simulink model "ASM_Traffic_V2X_Complete_Model_2"  (R2019a)
settings: Solver=ode1  StartTime=SIM.tstart.v  StopTime=Inf  FixedStep=SIM.StepSize.v  RelTol=1e-3
PostLoadFcn:
  | if any(exist('dsrtsu_mdlpostloadfcn', 'file') ~= 0), dsrtsu_mdlpostloadfcn('Execute', bdroot); end
  | try, asm_mdl_postloadfcn(bdroot, 'UpdateModel', 2200); catch, disp(lasterr); end,
undefined symbols (not defined in the file): _SensorPnts_1, _SensorPnts_13, _SensorPnts_17, _SensorPnts_21, _SensorPnts_25, _SensorPnts_29, _SensorPnts_33, _SensorPnts_37, _SensorPnts_41, _SensorPnts_45, _SensorPnts_49, _SensorPnts_5, _SensorPnts_53, _SensorPnts_57, _SensorPnts_9, _to_, CPT, G5A, ITS, MDL, rad, s_to_rpm, SIM
libraries: simulink x169, ASM_VehicleDynamics_lib x126, ASM_Traffic_lib x83, ASM_Utils_lib x49, mdbs x45, ASM_Environment_lib x17, dspindex x12, dsaV2xLibraryAux x10, dsmpblib x6, dsaV2xAsn1Library x4, dsaV2xLibrary x4, ASM_BrakeHydraulics_lib x4
(part 31 of 36)

== system ASM_Traffic_V2X_Complete_Model_2/MDLUserInterface/MotionDeskInterface/MOTION_DESK_INTERFACE/Traffic_Animation/Sensors_Animation/Sensor_Points/Line_Sensor_Junction_Shape_Line_Points ==
  ModelSignals : Inport
  Bus Selector : BusSelector  OutputSignals=Pos_x_Junction_Shape_Line_Animation_CoorSys_E,Pos_y_Junction_Shape_Line_Animation_CoorSys_E,Pos_z_Junction_Shape_Line_Animation_CoorSys_E
  CC : Concatenate  NumInputs=4  Mode=Multidimensional array
  Reshape1 : Reshape  OutputDimensionality=Row vector (2-D)
  Reshape2 : Reshape  OutputDimensionality=Row vector (2-D)
  Reshape3 : Reshape  OutputDimensionality=Row vector (2-D)
  zero : Constant  Value=zeros(1,60)  VectorParams1D=off
  AnimationSignals : Outport
  wires:
  zero/1 -> CC/4
  Reshape3/1 -> CC/3
  Reshape2/1 -> CC/2
  Reshape1/1 -> CC/1
  Bus Selector/3 -> Reshape3/1  "<Pos_z_Junction_Shape_Line_Animation_CoorSys_E>"
  Bus Selector/2 -> Reshape2/1  "<Pos_y_Junction_Shape_Line_Animation_CoorSys_E>"
  Bus Selector/1 -> Reshape1/1  "<Pos_x_Junction_Shape_Line_Animation_CoorSys_E>"
  CC/1 -> AnimationSignals/1
  ModelSignals/1 -> Bus Selector/1

== system ASM_Traffic_V2X_Complete_Model_2/MDLUserInterface/MotionDeskInterface/MOTION_DESK_INTERFACE/Traffic_Animation/Sensors_Animation/Sensor_Points/Line_Sensor_Road_Lane_Points ==
  ModelSignals : Inport
  Bus Selector : BusSelector  OutputSignals=Pos_x_Road_Lane_Animation_CoorSys_E,Pos_y_Road_Lane_Animation_CoorSys_E,Pos_z_Road_Lane_Animation_CoorSys_E
  CC : Concatenate  NumInputs=4  Mode=Multidimensional array
  Reshape1 : Reshape  OutputDimensionality=Row vector (2-D)
  Reshape2 : Reshape  OutputDimensionality=Row vector (2-D)
  Reshape3 : Reshape  OutputDimensionality=Row vector (2-D)
  zero : Constant  Value=zeros(1,60)  VectorParams1D=off
  AnimationSignals : Outport
  wires:
  Bus Selector/3 -> Reshape3/1  "<Pos_z_Road_Lane_Animation_CoorSys_E>"
  Bus Selector/2 -> Reshape2/1  "<Pos_y_Road_Lane_Animation_CoorSys_E>"
  Bus Selector/1 -> Reshape1/1  "<Pos_x_Road_Lane_Animation_CoorSys_E>"
  CC/1 -> AnimationSignals/1
  ModelSignals/1 -> Bus Selector/1
  Reshape1/1 -> CC/1
  Reshape2/1 -> CC/2
  Reshape3/1 -> CC/3
  zero/1 -> CC/4

== system ASM_Traffic_V2X_Complete_Model_2/MDLUserInterface/MotionDeskInterface/MOTION_DESK_INTERFACE/Traffic_Animation/Sensors_Animation/Sensor_Points/Line_Sensor_Road_Shape_ContObj_Points ==
  ModelSignals : Inport
  Bus Selector : BusSelector  OutputSignals=Pos_x_Road_Shape_ContObj_Animation_CoorSys_E,Pos_y_Road_Shape_ContObj_Animation_CoorSys_E,Pos_z_Road_Shape_ContObj_Animation_CoorSys_E
  CC : Concatenate  NumInputs=4  Mode=Multidimensional array
  Reshape1 : Reshape  OutputDimensionality=Row vector (2-D)
  Reshape2 : Reshape  OutputDimensionality=Row vector (2-D)
  Reshape3 : Reshape  OutputDimensionality=Row vector (2-D)
  zero : Constant  Value=zeros(1,60)  VectorParams1D=off
  AnimationSignals : Outport
  wires:
  ModelSignals/1 -> Bus Selector/1
  CC/1 -> AnimationSignals/1
  Bus Selector/1 -> Reshape1/1  "<Pos_x_Road_Shape_ContObj_Animation_CoorSys_E>"
  Bus Selector/2 -> Reshape2/1  "<Pos_y_Road_Shape_ContObj_Animation_CoorSys_E>"
  Bus Selector/3 -> Reshape3/1  "<Pos_z_Road_Shape_ContObj_Animation_CoorSys_E>"
  Reshape1/1 -> CC/1
  Reshape2/1 -> CC/2
  Reshape3/1 -> CC/3
  zero/1 -> CC/4

== system ASM_Traffic_V2X_Complete_Model_2/MDLUserInterface/MotionDeskInterface/MOTION_DESK_INTERFACE/Traffic_Animation/Sensors_Animation/Sensor_Points/Line_Sensor_Road_Shape_Line_Points ==
  ModelSignals : Inport
  Bus Selector : BusSelector  OutputSignals=Pos_x_Road_Shape_Line_Animation_CoorSys_E,Pos_y_Road_Shape_Line_Animation_CoorSys_E,Pos_z_Road_Shape_Line_Animation_CoorSys_E
  CC : Concatenate  NumInputs=4  Mode=Multidimensional array
  Reshape1 : Reshape  OutputDimensionality=Row vector (2-D)
  Reshape2 : Reshape  OutputDimensionality=Row vector (2-D)
  Reshape3 : Reshape  OutputDimensionality=Row vector (2-D)
  zero : Constant  Value=zeros(1,60)  VectorParams1D=off
  AnimationSignals : Outport
  wires:
  Bus Selector/3 -> Reshape3/1  "<Pos_z_Road_Shape_Line_Animation_CoorSys_E>"
  Bus Selector/2 -> Reshape2/1  "<Pos_y_Road_Shape_Line_Animation_CoorSys_E>"
  Bus Selector/1 -> Reshape1/1  "<Pos_x_Road_Shape_Line_Animation_CoorSys_E>"
  CC/1 -> AnimationSignals/1
  ModelSignals/1 -> Bus Selector/1
  Reshape1/1 -> CC/1
  Reshape2/1 -> CC/2
  Reshape3/1 -> CC/3
  zero/1 -> CC/4

== system ASM_Traffic_V2X_Complete_Model_2/MDLUserInterface/MotionDeskInterface/MOTION_DESK_INTERFACE/Traffic_Animation/Sensors_Animation/Sensor_Points/Object_Sensor_2D_Points ==
  Transform_In : Inport
  ModelSignals : Inport  Port=2
  Bus Selector1 : BusSelector  OutputSignals=Sensor_1_Front,Sensor_2_Front_Left,Sensor_3_Left,Sensor_4_Rear_Left,Sensor_5_Front_Right,Sensor_6_Right,Sensor_7_Rear_Right
  Bus Selector{2..8} (7 alike) : BusSelector  OutputSignals=Parameters.Pos_Sensor_Apex_CoorSys_V[x;y;z][m],Parameters.Angle_z_Orientation_Sensor_CoorSys_V[deg],SensorOutput.Angle_Hor_Rel[deg],SensorOutput.Distance[m],Parameters.Num_SensorRays_Used[],Parameters.Angle_ScopeZone_Horizontal[deg]  OutputAsBus=on
  Calc_Object_Sensor_2D_Points : Subsystem
  Multiport Switch : MultiPortSwitch  Inputs=7
  Object_Sensor_2D_Transformation : Subsystem
  Saturation : Saturate  UpperLimit=7  LowerLimit=1
  Sensor_Selector : Constant
  AnimationSignals : Outport
  wires:
  Saturation/1 -> Multiport Switch/1
  Bus Selector1/7 -> Bus Selector8/1  "<Sensor_7_Rear_Right>"
  Bus Selector1/6 -> Bus Selector5/1  "<Sensor_6_Right>"
  Bus Selector1/5 -> Bus Selector3/1  "<Sensor_5_Front_Right>"
  Bus Selector1/4 -> Bus Selector2/1  "<Sensor_4_Rear_Left>"
  Bus Selector8/1 -> Multiport Switch/8
  Bus Selector5/1 -> Multiport Switch/7
  Bus Selector3/1 -> Multiport Switch/6
  Bus Selector2/1 -> Multiport Switch/5
  Transform_In/1 -> Object_Sensor_2D_Transformation/1(Transform_In1)
  Object_Sensor_2D_Transformation/1(Transform_Out) -> Calc_Object_Sensor_2D_Points/1(Transform_In)
  Calc_Object_Sensor_2D_Points/1(AnimationSignals) -> AnimationSignals/1
  ModelSignals/1 -> Bus Selector1/1
  Bus Selector1/1 -> Bus Selector4/1  "<Sensor_1_Front>"
  Bus Selector1/2 -> Bus Selector6/1  "<Sensor_2_Front_Left>"
  Bus Selector1/3 -> Bus Selector7/1  "<Sensor_3_Left>"
  Bus Selector7/1 -> Multiport Switch/4
  Bus Selector6/1 -> Multiport Switch/3
  Bus Selector4/1 -> Multiport Switch/2
  Sensor_Selector/1 -> Saturation/1
  Multiport Switch/1 -> Calc_Object_Sensor_2D_Points/2(ModelSignals), Object_Sensor_2D_Transformation/2(ModelSignals)

== system ASM_Traffic_V2X_Complete_Model_2/MDLUserInterface/MotionDeskInterface/MOTION_DESK_INTERFACE/Traffic_Animation/Sensors_Animation/Sensor_Points/Object_Sensor_3D_CustomPoints ==
  ModelSignals : Inport
  Sensor_Selector : Inport  Port=2
  AdaptPointSensor1_To_Dim_60 : Subsystem
  AdaptPointSensor2_To_Dim_60 : Subsystem
  AdaptPointSensor3_To_Dim_60 : Subsystem
  Bus Selector1 : BusSelector  OutputSignals=Sensor_1_Front_Long,Sensor_2_Front_Mid,Sensor_3_Rear
  Bus Selector3 : BusSelector  OutputSignals=ID[],Pos_CoorSys_E[x;y;z][m]
  Bus Selector4 : BusSelector  OutputSignals=CustomPoints.ID[],CustomPoints.Pos_CoorSys_E[x;y;z][m]  OutputAsBus=on
  Bus Selector5 : BusSelector  OutputSignals=ID[],Pos_CoorSys_E[x;y;z][m]
  Bus Selector6 : BusSelector  OutputSignals=CustomPoints.ID[],CustomPoints.Pos_CoorSys_E[x;y;z][m]  OutputAsBus=on
  Bus Selector7 : BusSelector  OutputSignals=CustomPoints.ID[],CustomPoints.Pos_CoorSys_E[x;y;z][m]  OutputAsBus=on
  Bus Selector8 : BusSelector  OutputSignals=ID[],Pos_CoorSys_E[x;y;z][m]
  Compare To Constant3 : simulink/Logic and Bit Operations/Compare To Constant  relop=>  const=-1  OutDataTypeStr=boolean
  DownAway_Dim_3_60 : Constant  Value=[zeros(60*2,1); zeros(60,1)-999999]
  Multiport Switch1 : MultiPortSwitch
  Multiport Switch2 : MultiPortSwitch
  Mux : Mux  Inputs=3
  Reshape_60_3 : Reshape  OutputDimensionality=Customize  OutputDimensions=[60,3]
  Saturation1 : Saturate  UpperLimit=3  LowerLimit=1
  Sw : MultiPortSwitch  DataPortOrder=Zero-based contiguous  Inputs=2  zeroidx=on
  Transpose : Math  Operator=transpose  SaturateOnIntegerOverflow=on
  cc1 : Concatenate  Mode=Multidimensional array
  zero_60 : Constant  Value=zeros(1,60)  VectorParams1D=off
  AnimationSignals : Outport
  wires:
  cc1/1 -> AnimationSignals/1
  zero_60/1 -> cc1/2
  AdaptPointSensor3_To_Dim_60/1(ID_Adatpted[]) -> Multiport Switch2/4
  AdaptPointSensor3_To_Dim_60/2(Pos_ObjectPoint_CoorSys_E_Adapted[x;y;z][m]) -> Multiport Switch1/4
  Multiport Switch1/1 -> Sw/3
  Bus Selector8/2 -> AdaptPointSensor3_To_Dim_60/2(Pos_ObjectPoint_CoorSys_E[x;y;z][m])  "<Pos_CoorSys_E[x;y;z][m]>"
  Bus Selector5/2 -> AdaptPointSensor2_To_Dim_60/2(Pos_ObjectPoint_CoorSys_E[x;y;z][m])  "<Pos_CoorSys_E[x;y;z][m]>"
  Bus Selector5/1 -> AdaptPointSensor2_To_Dim_60/1(ID[])  "<ID[]>"
  Bus Selector1/1 -> Bus Selector4/1  "<Sensor_1_Front_Long>"
  Bus Selector1/2 -> Bus Selector6/1  "<Sensor_2_Front_Mid>"
  Bus Selector1/3 -> Bus Selector7/1  "<Sensor_3_Rear>"
  Multiport Switch2/1 -> Compare To Constant3/1
  Reshape_60_3/1 -> Transpose/1
  Bus Selector6/1 -> Bus Selector5/1
  Bus Selector7/1 -> Bus Selector8/1
  Bus Selector3/1 -> AdaptPointSensor1_To_Dim_60/1(ID[])  "<ID[]>"
  Bus Selector3/2 -> AdaptPointSensor1_To_Dim_60/2(Pos_ObjectPoint_CoorSys_E[x;y;z][m])  "<Pos_CoorSys_E[x;y;z][m]>"
  Bus Selector4/1 -> Bus Selector3/1
  AdaptPointSensor1_To_Dim_60/1(ID_Adatpted[]) -> Multiport Switch2/2
  AdaptPointSensor1_To_Dim_60/2(Pos_ObjectPoint_CoorSys_E_Adapted[x;y;z][m]) -> Multiport Switch1/2
  Bus Selector8/1 -> AdaptPointSensor3_To_Dim_60/1(ID[])  "<ID[]>"
  ModelSignals/1 -> Bus Selector1/1
  Mux/1 -> Sw/1
  Compare To Constant3/1 -> Mux/3, Mux/2, Mux/1
  Sensor_Selector/1 -> Saturation1/1
  DownAway_Dim_3_60/1 -> Sw/2
  Saturation1/1 -> Multiport Switch1/1, Multiport Switch2/1
  Sw/1 -> Reshape_60_3/1
  Transpose/1 -> cc1/1
  AdaptPointSensor2_To_Dim_60/2(Pos_ObjectPoint_CoorSys_E_Adapted[x;y;z][m]) -> Multiport Switch1/3
  AdaptPointSensor2_To_Dim_60/1(ID_Adatpted[]) -> Multiport Switch2/3

== system ASM_Traffic_V2X_Complete_Model_2/MDLUserInterface/MotionDeskInterface/MOTION_DESK_INTERFACE/Traffic_Animation/Sensors_Animation/Sensor_Points/Object_Sensor_3D_Points ==
  ModelSignals : Inport
  Sensor_Selector : Inport  Port=2
  Bus Selector1 : BusSelector  OutputSignals=Sensor_1_Front_Long,Sensor_2_Front_Mid,Sensor_3_Rear
  Bus Selector2 : BusSelector  OutputSignals=Flag_NearestPnt_Occluded[-1|0|1],Flag_Object_In_Scope[0Out|1In],Pos_Object_NearestPnt_E[x;y;z][m]
  Bus Selector4 : BusSelector  OutputSignals=SensorOutput.Pos_Object_NearestPnt_E[x;y;z][m],Info.Flag_Object_In_Scope[0Out|1In],SensorOutput.Flag_NearestPnt_Occluded[-1|0|1]  OutputAsBus=on
  Bus Selector6 : BusSelector  OutputSignals=SensorOutput.Pos_Object_NearestPnt_E[x;y;z][m],Info.Flag_Object_In_Scope[0Out|1In],SensorOutput.Flag_NearestPnt_Occluded[-1|0|1]  OutputAsBus=on
  Bus Selector7 : BusSelector  OutputSignals=SensorOutput.Pos_Object_NearestPnt_E[x;y;z][m],Info.Flag_Object_In_Scope[0Out|1In],SensorOutput.Flag_NearestPnt_Occluded[-1|0|1]  OutputAsBus=on
  DownAway : Constant  Value=[zeros(MDL.Traffic.Sensors.ObjectSensor3D_Calculation.Const_Sensor_Output_Dimension.v*2,1); zeros(MDL.Traffic.Sensors.ObjectSensor3D_Calculation.Const_Sensor_Output_Dimension.v,1)-999999]
  DownAway1 : Constant  Value=[zeros(2,60-MDL.Traffic.Sensors.ObjectSensor3D_Calculation.Const_Sensor_Output_Dimension.v); zeros(1,60-MDL.Traffic.Sensors.ObjectSensor3D_Calculation.Const_Sensor_Output_Dimension.v)-999999]
  Hide_Occluded_NearestPoint[0|1] : Constant  Value=0
  Ignore_Negative : RelationalOperator  Operator===  RndMeth=Simplest
  Mask_Hidden_Objects : Product
  Multiport Switch : MultiPortSwitch
  Mux : Mux  Inputs=3
  Negate : Sum  Inputs=+-
  Product : Product
  Reshape1 : Reshape  OutputDimensionality=Customize  OutputDimensions=[MDL.Traffic.Sensors.ObjectSensor3D_Calculation.Const_Sensor_Output_Dimension.v,3]
  Saturation : Saturate  UpperLimit=3  LowerLimit=1
  Saturation1 : Saturate  UpperLimit=1  LowerLimit=0
  Show_Occluded_NearestPoint[0|1]1 : Constant
  Show_Occluded_NearestPoint[0|1]2 : Constant
  Sw : MultiPortSwitch  DataPortOrder=Zero-based contiguous  Inputs=2  zeroidx=on
  Transpose : Math  Operator=transpose  SaturateOnIntegerOverflow=on
  cc : Concatenate  Mode=Multidimensional array  ConcatenateDimension=2
  cc1 : Concatenate  Mode=Multidimensional array
  zero3 : Constant  Value=zeros(1,60)  VectorParams1D=off
  AnimationSignals : Outport
  wires:
  Mask_Hidden_Objects/1 -> Mux/2, Mux/1, Mux/3
  Negate/1 -> Mask_Hidden_Objects/1
  Bus Selector2/2 -> Mask_Hidden_Objects/2  "<Flag_Object_In_Scope[0Out|1In]>"
  Ignore_Negative/1 -> Product/2
  Show_Occluded_NearestPoint[0|1]2/1 -> Ignore_Negative/2
  Bus Selector2/1 -> Ignore_Negative/1  "<Flag_NearestPnt_Occluded[-1|0|1]>"
  Show_Occluded_NearestPoint[0|1]1/1 -> Negate/1
  Product/1 -> Negate/2
  Mux/1 -> Sw/1
  Saturation1/1 -> Product/1
  Hide_Occluded_NearestPoint[0|1]/1 -> Saturation1/1
  Saturation/1 -> Multiport Switch/1
  ModelSignals/1 -> Bus Selector1/1
  Bus Selector1/1 -> Bus Selector4/1  "<Sensor_1_Front_Long>"
  Bus Selector1/2 -> Bus Selector6/1  "<Sensor_2_Front_Mid>"
  Bus Selector1/3 -> Bus Selector7/1  "<Sensor_3_Rear>"
  Bus Selector7/1 -> Multiport Switch/4
  Bus Selector6/1 -> Multiport Switch/3
  Bus Selector4/1 -> Multiport Switch/2
  Sensor_Selector/1 -> Saturation/1
  Multiport Switch/1 -> Bus Selector2/1
  Bus Selector2/3 -> Sw/3  "<Pos_Object_NearestPnt_E[x;y;z][m]>"
  DownAway/1 -> Sw/2
  Sw/1 -> Reshape1/1
  Reshape1/1 -> Transpose/1
  Transpose/1 -> cc/1
  DownAway1/1 -> cc/2
  cc/1 -> cc1/1
  zero3/1 -> cc1/2
  cc1/1 -> AnimationSignals/1

== system ASM_Traffic_V2X_Complete_Model_2/MDLUserInterface/MotionDeskInterface/MOTION_DESK_INTERFACE/Traffic_Animation/Sensors_Animation/Sensor_Points/Object_Sensor_3D_RadarEffect_Points ==
  ModelSignals : Inport
  Sensor_Selector : Inport  Port=2
  AdaptPointDimensionSensor1 : Subsystem
  AdaptPointDimensionSensor2 : Subsystem
  AdaptPointDimensionSensor3 : Subsystem
  Bus Selector1 : BusSelector  OutputSignals=Sensor_1_Front_Long,Sensor_2_Front_Mid,Sensor_3_Rear
  Bus Selector3 : BusSelector  OutputSignals=ID[],Pos_ObjectPoint_CoorSys_E[x;y;z][m]
  Bus Selector4 : BusSelector  OutputSignals=RadarEffects.ID[],RadarEffects.Pos_ObjectPoint_CoorSys_E[x;y;z][m]  OutputAsBus=on
  Bus Selector5 : BusSelector  OutputSignals=ID[],Pos_ObjectPoint_CoorSys_E[x;y;z][m]
  Bus Selector6 : BusSelector  OutputSignals=RadarEffects.ID[],RadarEffects.Pos_ObjectPoint_CoorSys_E[x;y;z][m]  OutputAsBus=on
  Bus Selector7 : BusSelector  OutputSignals=RadarEffects.ID[],RadarEffects.Pos_ObjectPoint_CoorSys_E[x;y;z][m]  OutputAsBus=on
  Bus Selector8 : BusSelector  OutputSignals=ID[],Pos_ObjectPoint_CoorSys_E[x;y;z][m]
  Compare To Constant3 : simulink/Logic and Bit Operations/Compare To Constant  relop=>  const=-1  OutDataTypeStr=boolean
  DownAway : Constant  Value=[zeros(60*2,1); zeros(60,1)-999999]
  Multiport Switch1 : MultiPortSwitch
  Multiport Switch2 : MultiPortSwitch
  Mux : Mux  Inputs=3
  Reshape1 : Reshape  OutputDimensionality=Customize  OutputDimensions=[60,3]
  Saturation1 : Saturate  UpperLimit=3  LowerLimit=1
  Sw : MultiPortSwitch  DataPortOrder=Zero-based contiguous  Inputs=2  zeroidx=on
  Transpose : Math  Operator=transpose  SaturateOnIntegerOverflow=on
  cc1 : Concatenate  Mode=Multidimensional array
  zero3 : Constant  Value=zeros(1,60)  VectorParams1D=off
  AnimationSignals : Outport
  wires:
  Bus Selector8/2 -> AdaptPointDimensionSensor3/2(Pos_ObjectPoint_CoorSys_E[x;y;z][m])  "<Pos_ObjectPoint_CoorSys_E[x;y;z][m]>"
  cc1/1 -> AnimationSignals/1
  zero3/1 -> cc1/2
  Transpose/1 -> cc1/1
  Reshape1/1 -> Transpose/1
  Mux/1 -> Sw/1
  Sw/1 -> Reshape1/1
  DownAway/1 -> Sw/2
  Compare To Constant3/1 -> Mux/1, Mux/2, Mux/3
  AdaptPointDimensionSensor3/2(Pos_ObjectPoint_CoorSys_E_Adapted[x;y;z][m]) -> Multiport Switch1/4
  AdaptPointDimensionSensor3/1(ID_Adatpted[]) -> Multiport Switch2/4
  Bus Selector5/2 -> AdaptPointDimensionSensor2/2(Pos_ObjectPoint_CoorSys_E[x;y;z][m])  "<Pos_ObjectPoint_CoorSys_E[x;y;z][m]>"
  AdaptPointDimensionSensor2/2(Pos_ObjectPoint_CoorSys_E_Adapted[x;y;z][m]) -> Multiport Switch1/3
  AdaptPointDimensionSensor2/1(ID_Adatpted[]) -> Multiport Switch2/3
  AdaptPointDimensionSensor1/2(Pos_ObjectPoint_CoorSys_E_Adapted[x;y;z][m]) -> Multiport Switch1/2
  AdaptPointDimensionSensor1/1(ID_Adatpted[]) -> Multiport Switch2/2
  Bus Selector3/2 -> AdaptPointDimensionSensor1/2(Pos_ObjectPoint_CoorSys_E[x;y;z][m])  "<Pos_ObjectPoint_CoorSys_E[x;y;z][m]>"
  Bus Selector3/1 -> AdaptPointDimensionSensor1/1(ID[])  "<ID[]>"
  Multiport Switch1/1 -> Sw/3
  Multiport Switch2/1 -> Compare To Constant3/1
  Bus Selector8/1 -> AdaptPointDimensionSensor3/1(ID[])  "<ID[]>"
  Bus Selector5/1 -> AdaptPointDimensionSensor2/1(ID[])  "<ID[]>"
  Sensor_Selector/1 -> Saturation1/1
  Saturation1/1 -> Multiport Switch2/1, Multiport Switch1/1
  ModelSignals/1 -> Bus Selector1/1
  Bus Selector1/1 -> Bus Selector4/1  "<Sensor_1_Front_Long>"
  Bus Selector1/2 -> Bus Selector6/1  "<Sensor_2_Front_Mid>"
  Bus Selector1/3 -> Bus Selector7/1  "<Sensor_3_Rear>"
  Bus Selector7/1 -> Bus Selector8/1
  Bus Selector6/1 -> Bus Selector5/1
  Bus Selector4/1 -> Bus Selector3/1

== system ASM_Traffic_V2X_Complete_Model_2/MDLUserInterface/MotionDeskInterface/MOTION_DESK_INTERFACE/Traffic_Animation/Sensors_Animation/Sensor_Points/Sensor_Points ==
  AnimationSignals : Inport
  MD_Object1 : mdbs/MD_Object  strObjId=23  strObjName=_SensorPnts_1-4  strBlockType=OBJ  bGUIEventOK=0
      settings: SourceProductName=dSPACE MotionDesk Blockset
  MD_Object10 : mdbs/MD_Object  strObjId=32  strObjName=_SensorPnts_37-40  strBlockType=OBJ  bGUIEventOK=0
      settings: SourceProductName=dSPACE MotionDesk Blockset
  MD_Object11 : mdbs/MD_Object  strObjId=35  strObjName=_SensorPnts_49-52  strBlockType=OBJ  bGUIEventOK=0
      settings: SourceProductName=dSPACE MotionDesk Blockset
  MD_Object13 : mdbs/MD_Object  strObjId=33  strObjName=_SensorPnts_41-44  strBlockType=OBJ  bGUIEventOK=0
      settings: SourceProductName=dSPACE MotionDesk Blockset
  MD_Object14 : mdbs/MD_Object  strObjId=34  strObjName=_SensorPnts_45-48  strBlockType=OBJ  bGUIEventOK=0
      settings: SourceProductName=dSPACE MotionDesk Blockset
  MD_Object15 : mdbs/MD_Object  strObjId=36  strObjName=_SensorPnts_53-56  strBlockType=OBJ  bGUIEventOK=0
      settings: SourceProductName=dSPACE MotionDesk Blockset
  MD_Object16 : mdbs/MD_Object  strObjId=37  strObjName=_SensorPnts_57-60  strBlockType=OBJ  bGUIEventOK=0
      settings: SourceProductName=dSPACE MotionDesk Blockset
  MD_Object2 : mdbs/MD_Object  strObjId=24  strObjName=_SensorPnts_5-8  strBlockType=OBJ  bGUIEventOK=0
      settings: SourceProductName=dSPACE MotionDesk Blockset
  MD_Object3 : mdbs/MD_Object  strObjId=25  strObjName=_SensorPnts_9-12  strBlockType=OBJ  bGUIEventOK=0
      settings: SourceProductName=dSPACE MotionDesk Blockset
  MD_Object4 : mdbs/MD_Object  strObjId=26  strObjName=_SensorPnts_13-16  strBlockType=OBJ  bGUIEventOK=0
      settings: SourceProductName=dSPACE MotionDesk Blockset
  MD_Object5 : mdbs/MD_Object  strObjId=27  strObjName=_SensorPnts_17-20  strBlockType=OBJ  bGUIEventOK=0
      settings: SourceProductName=dSPACE MotionDesk Blockset
  MD_Object6 : mdbs/MD_Object  strObjId=28  strObjName=_SensorPnts_21-24  strBlockType=OBJ  bGUIEventOK=0
      settings: SourceProductName=dSPACE MotionDesk Blockset
  MD_Object7 : mdbs/MD_Object  strObjId=29  strObjName=_SensorPnts_25-28  strBlockType=OBJ  bGUIEventOK=0
      settings: SourceProductName=dSPACE MotionDesk Blockset
  MD_Object8 : mdbs/MD_Object  strObjId=30  strObjName=_SensorPnts_29-32  strBlockType=OBJ  bGUIEventOK=0
      settings: SourceProductName=dSPACE MotionDesk Blockset
  MD_Object9 : mdbs/MD_Object  strObjId=31  strObjName=_SensorPnts_33-36  strBlockType=OBJ  bGUIEventOK=0
      settings: SourceProductName=dSPACE MotionDesk Blockset
  Selector : Selector  NumberOfDimensions=2  IndexMode=Zero-based  InputPortWidth=15  IndexOptions=Index vector (dialog),Index vector (dialog)  Indices=-1,[0:3]  OutputSizes=1,1
  Selector1 : Selector  NumberOfDimensions=2  IndexMode=Zero-based  InputPortWidth=15  IndexOptions=Index vector (dialog),Index vector (dialog)  Indices=-1,[0:3]+4  OutputSizes=1,1
  Selector10 : Selector  NumberOfDimensions=2  IndexMode=Zero-based  InputPortWidth=15  IndexOptions=Index vector (dialog),Index vector (dialog)  Indices=-1,[0:3]+52  OutputSizes=1,1
  Selector12 : Selector  NumberOfDimensions=2  IndexMode=Zero-based  InputPortWidth=15  IndexOptions=Index vector (dialog),Index vector (dialog)  Indices=-1,[0:3]+40  OutputSizes=1,1
  Selector13 : Selector  NumberOfDimensions=2  IndexMode=Zero-based  InputPortWidth=15  IndexOptions=Index vector (dialog),Index vector (dialog)  Indices=-1,[0:3]+44  OutputSizes=1,1
  Selector14 : Selector  NumberOfDimensions=2  IndexMode=Zero-based  InputPortWidth=15  IndexOptions=Index vector (dialog),Index vector (dialog)  Indices=-1,[0:3]+56  OutputSizes=1,1
  Selector15 : Selector  NumberOfDimensions=2  IndexMode=Zero-based  InputPortWidth=15  IndexOptions=Index vector (dialog),Index vector (dialog)  Indices=-1,[0:3]+48  OutputSizes=1,1
  Selector2 : Selector  NumberOfDimensions=2  IndexMode=Zero-based  InputPortWidth=15  IndexOptions=Index vector (dialog),Index vector (dialog)  Indices=-1,[0:3]+8  OutputSizes=1,1
  Selector3 : Selector  NumberOfDimensions=2  IndexMode=Zero-based  InputPortWidth=15  IndexOptions=Index vector (dialog),Index vector (dialog)  Indices=-1,[0:3]+12  OutputSizes=1,1
  Selector4 : Selector  NumberOfDimensions=2  IndexMode=Zero-based  InputPortWidth=15  IndexOptions=Index vector (dialog),Index vector (dialog)  Indices=-1,[0:3]+16  OutputSizes=1,1
  Selector5 : Selector  NumberOfDimensions=2  IndexMode=Zero-based  InputPortWidth=15  IndexOptions=Index vector (dialog),Index vector (dialog)  Indices=-1,[0:3]+20  OutputSizes=1,1
  Selector6 : Selector  NumberOfDimensions=2  IndexMode=Zero-based  InputPortWidth=15  IndexOptions=Index vector (dialog),Index vector (dialog)  Indices=-1,[0:3]+24  OutputSizes=1,1
  Selector7 : Selector  NumberOfDimensions=2  IndexMode=Zero-based  InputPortWidth=15  IndexOptions=Index vector (dialog),Index vector (dialog)  Indices=-1,[0:3]+28  OutputSizes=1,1
  Selector8 : Selector  NumberOfDimensions=2  IndexMode=Zero-based  InputPortWidth=15  IndexOptions=Index vector (dialog),Index vector (dialog)  Indices=-1,[0:3]+32  OutputSizes=1,1
  Selector9 : Selector  NumberOfDimensions=2  IndexMode=Zero-based  InputPortWidth=15  IndexOptions=Index vector (dialog),Index vector (dialog)  Indices=-1,[0:3]+36  OutputSizes=1,1
  Terminator{1..11,13..16} (15 alike) : Terminator
  wires:
  Selector8/1 -> MD_Object9/1
  Selector7/1 -> MD_Object8/1
  Selector6/1 -> MD_Object7/1
  Selector5/1 -> MD_Object6/1
  Selector4/1 -> MD_Object5/1
  Selector3/1 -> MD_Object4/1
  MD_Object9/1 -> Terminator9/1
  Selector2/1 -> MD_Object3/1
  Selector1/1 -> MD_Object2/1
  Selector/1 -> MD_Object1/1
  MD_Object8/1 -> Terminator8/1
  MD_Object7/1 -> Terminator7/1
  MD_Object6/1 -> Terminator6/1
  MD_Object5/1 -> Terminator5/1
  MD_Object4/1 -> Terminator4/1
  MD_Object3/1 -> Terminator3/1
  MD_Object2/1 -> Terminator2/1
  MD_Object1/1 -> Terminator1/1
  MD_Object10/1 -> Terminator10/1
  Selector9/1 -> MD_Object10/1
  MD_Object13/1 -> Terminator13/1
  Selector12/1 -> MD_Object13/1
  MD_Object14/1 -> Terminator14/1
  Selector13/1 -> MD_Object14/1
  AnimationSignals/1 -> Selector/1, Selector15/1, Selector10/1, Selector14/1, Selector13/1, Selector12/1, Selector9/1, Selector8/1, Selector7/1, Selector6/1, Selector5/1, Selector4/1, Selector3/1, Selector2/1, Selector1/1
  MD_Object15/1 -> Terminator11/1
  Selector10/1 -> MD_Object15/1
  MD_Object16/1 -> Terminator15/1
  Selector14/1 -> MD_Object16/1
  Selector15/1 -> MD_Object11/1
  MD_Object11/1 -> Terminator16/1

== system ASM_Traffic_V2X_Complete_Model_2/MDLUserInterface/MotionDeskInterface/MOTION_DESK_INTERFACE/Traffic_Animation/Sensors_Animation/Sensor_Points/Traffic_Sign_Sensor_Points ==
  ModelSignals : Inport
  Bus Selector2 : BusSelector  OutputSignals=Sensor_Front_1.SensorOutput[].Traffic_Sign_Valid[0|1],Sensor_Front_1.SensorOutput[].Pos_CoorSys_E[x;y;z][m]
  DownAway : Constant  Value=[zeros(2,MDL.Traffic.Sensors.TrafficSignSensorDyn_Calculation.Const_Sensor_Output_Dimension.v); zeros(1,MDL.Traffic.Sensors.TrafficSignSensorDyn_Calculation.Const_Sensor_Output_Dimension.v)-999999]
  DownAway1 : Constant  Value=[zeros(2,60-MDL.Traffic.Sensors.TrafficSignSensorDyn_Calculation.Const_Sensor_Output_Dimension.v); zeros(1,60-MDL.Traffic.Sensors.TrafficSignSensorDyn_Calculation.Const_Sensor_Output_Dimension.v)-999999]
  Reshape1 : Reshape  OutputDimensionality=Customize  OutputDimensions=[3,MDL.Traffic.Sensors.TrafficSignSensorDyn_Calculation.Const_Sensor_Output_Dimension.v]
  Sw : MultiPortSwitch  DataPortOrder=Zero-based contiguous  Inputs=2  zeroidx=on
  Trans : Math  Operator=transpose  SaturateOnIntegerOverflow=on
  cc : Concatenate  NumInputs=3  Mode=Multidimensional array  ConcatenateDimension=2
  cc1 : Concatenate  Mode=Multidimensional array  ConcatenateDimension=2
  cc2 : Concatenate  Mode=Multidimensional array
  zero3 : Constant  Value=zeros(1,60)  VectorParams1D=off
  AnimationSignals : Outport
  wires:
  cc2/1 -> AnimationSignals/1
  cc1/1 -> cc2/1
  zero3/1 -> cc2/2
  Sw/1 -> cc1/1
  DownAway1/1 -> cc1/2
  DownAway/1 -> Sw/2
  Trans/1 -> Sw/1
  cc/1 -> Trans/1
  Reshape1/1 -> Sw/3
  Bus Selector2/1 -> cc/2, cc/1, cc/3  "<Traffic_Sign_Valid[0|1]>"
  Bus Selector2/2 -> Reshape1/1  "<Pos_CoorSys_E[x;y;z][m]>"
  ModelSignals/1 -> Bus Selector2/1

== system ASM_Traffic_V2X_Complete_Model_2/IO/I//O_Subsystem/Bus Configuration (1) - In/Simulated ECUs/DrivekitCAN/Drivekit/TX/PDUs ==
  Input : Inport
  BRAKE_REPORT : Subsystem
  Bus Selector : BusSelector  OutputSignals=signal3.Lat Value,signal3.Long Value,signal3.Heading Value,CurrentLane
  CHASSIS_CONTROL_REPORT : Subsystem
  ESP12 : Subsystem
  FAULT_REPORT : Subsystem
  GPS_HEADING : Subsystem
  GPS_LAT : Subsystem
  GPS_LONG : Subsystem
  LANE_REPORT : Subsystem
  SAS11 : Subsystem
  STEERING_ANGLE_REPORT : Subsystem
  STEERING_REPORT : Subsystem
  THROTTLE_REPORT : Subsystem
  WHL_SPD11 : Subsystem
  _PDUs_ : BusCreator  Inputs=13
  PDUs : Outport
  wires:
  _PDUs_/1 -> PDUs/1  "PDUs"
  SAS11/1(SAS11) -> _PDUs_/1  "SAS11"
  WHL_SPD11/1(WHL_SPD11) -> _PDUs_/2  "WHL_SPD11"
  ESP12/1(ESP12) -> _PDUs_/3  "ESP12"
  BRAKE_REPORT/1(BRAKE_REPORT) -> _PDUs_/4  "BRAKE_REPORT"
  STEERING_REPORT/1(STEERING_REPORT) -> _PDUs_/5  "STEERING_REPORT"
  THROTTLE_REPORT/1(THROTTLE_REPORT) -> _PDUs_/6  "THROTTLE_REPORT"
  FAULT_REPORT/1(FAULT_REPORT) -> _PDUs_/7  "FAULT_REPORT"
  STEERING_ANGLE_REPORT/1(STEERING_ANGLE_REPORT) -> _PDUs_/8  "STEERING_ANGLE_REPORT"
  CHASSIS_CONTROL_REPORT/1(CHASSIS_CONTROL_REPORT) -> _PDUs_/9  "CHASSIS_CONTROL_REPORT"
  GPS_LAT/1(GPS_LAT) -> _PDUs_/10  "GPS_LAT"
  GPS_LONG/1(GPS_LONG) -> _PDUs_/11  "GPS_LONG"
  GPS_HEADING/1(GPS_HEADING) -> _PDUs_/12  "GPS_HEADING"
  LANE_REPORT/1(LANE_REPORT) -> _PDUs_/13  "LANE_REPORT"
  Input/1 -> SAS11/1(Input), Bus Selector/1, WHL_SPD11/1(Input)
  Bus Selector/1 -> GPS_LAT/1(Input)  "<Lat Value>"
  Bus Selector/2 -> GPS_LONG/1(Input)  "<Long Value>"
  Bus Selector/3 -> GPS_HEADING/1(Input)  "<Heading Value>"
  Bus Selector/4 -> LANE_REPORT/1(Input)  "<CurrentLane>"

== system ASM_Traffic_V2X_Complete_Model_2/IO/I//O_Subsystem/Bus Configuration (1) - Out/Simulated ECUs/DrivekitCAN/Drivekit/RX/PDUs ==
  PDUs : Inport
  BRAKE_COMMAND : Subsystem
  BRAKE_DISABLE : Subsystem
  BRAKE_ENABLE : Subsystem
  CHASSIS_CONTROL_COMMAND : Subsystem
  STEERING_ANGLE_COMMAND : Subsystem
  STEERING_DISABLE : Subsystem
  STEERING_ENABLE : Subsystem
  STEERING_TORQUE_COMMAND : Subsystem
  THROTTLE_COMMAND : Subsystem
  THROTTLE_DISABLE : Subsystem
  THROTTLE_ENABLE : Subsystem
  _PDUs_ : BusSelector  OutputSignals=BRAKE_ENABLE,BRAKE_DISABLE,BRAKE_COMMAND,STEERING_ENABLE,STEERING_DISABLE,STEERING_TORQUE_COMMAND,THROTTLE_ENABLE,THROTTLE_DISABLE,THROTTLE_COMMAND,STEERING_ANGLE_COMMAND,CHASSIS_CONTROL_COMMAND
  wires:
  PDUs/1 -> _PDUs_/1  "PDUs"
  _PDUs_/1 -> BRAKE_ENABLE/1(BRAKE_ENABLE)  "<BRAKE_ENABLE>"
  _PDUs_/2 -> BRAKE_DISABLE/1(BRAKE_DISABLE)  "<BRAKE_DISABLE>"
  _PDUs_/3 -> BRAKE_COMMAND/1(BRAKE_COMMAND)  "<BRAKE_COMMAND>"
  _PDUs_/4 -> STEERING_ENABLE/1(STEERING_ENABLE)  "<STEERING_ENABLE>"
  _PDUs_/5 -> STEERING_DISABLE/1(STEERING_DISABLE)  "<STEERING_DISABLE>"
  _PDUs_/6 -> STEERING_TORQUE_COMMAND/1(STEERING_TORQUE_COMMAND)  "<STEERING_TORQUE_COMMAND>"
  _PDUs_/7 -> THROTTLE_ENABLE/1(THROTTLE_ENABLE)  "<THROTTLE_ENABLE>"
  _PDUs_/8 -> THROTTLE_DISABLE/1(THROTTLE_DISABLE)  "<THROTTLE_DISABLE>"
  _PDUs_/9 -> THROTTLE_COMMAND/1(THROTTLE_COMMAND)  "<THROTTLE_COMMAND>"
  _PDUs_/10 -> STEERING_ANGLE_COMMAND/1(STEERING_ANGLE_COMMAND)  "<STEERING_ANGLE_COMMAND>"
  _PDUs_/11 -> CHASSIS_CONTROL_COMMAND/1(CHASSIS_CONTROL_COMMAND)  "<CHASSIS_CONTROL_COMMAND>"

== system ASM_Traffic_V2X_Complete_Model_2/MDL/Environment/Traffic/Sensors/Object_Sensor_3D/CustomPoints/Sensor1/CustomPoints ==
  Sensor_Idx[] : Inport
  Sensor_Data[] : Inport  Port=2
  Enable : EnablePort
  Bus Creator2 : BusCreator  Inputs=17
  CUSTOM_POINTS_1 : ASM_Traffic_lib/Sensors/Custom Points/CUSTOM_POINTS  Tag=ASM_SUBCOMPONENT  Sw_Visible_Points_Filter_Enable=MDL.Traffic.Sensors.CustomPoints_1.Sw_Visible_Points_Filter_Enable  Sw_Sort_Enable=MDL.Traffic.Sensors.CustomPoints_1.Sw_Sort_Enable  Sw_Sort_Attribute=MDL.Traffic.Sensors.CustomPoints_1.Sw_Sort_Attribute  Sw_Sort_Direction=MDL.Traffic.Sensors.CustomPoints_1.Sw_Sort_Direction  ASMProperties=struct('Name','CUSTOM_POINTS','Version','1.0','Library','ASM_Traffic_lib')  ASMInstanceName=custom_points  ASMInstanceID=1  Const_Output_Dimension_Objects=MDL.Traffic.Sensors.CustomPoints_1.Const_Output_Dimension_Objects  Const_Output_Dimension_Object_Points=MDL.Traffic.Sensors.CustomPoints_1.Const_Output_Dimension_Object_Points
  MODELDESK_GROUP : ASM_Utils_lib/ModelDeskInterface/MODELDESK_GROUP  MDLDGroup=Object Sensor 3D 1  ASMProperties=struct('Name','MODELDESK_GROUP','Version','1.0','Library','ASM_Utils_lib')
  Terminator : Terminator
  CustomPoint_Signals[] : Outport  OutputWhenDisabled=reset  InitialOutput=[0]
  wires:
  CUSTOM_POINTS_1/18 -> Bus Creator2/17  "Object_Type[]"
  CUSTOM_POINTS_1/7 -> Bus Creator2/6  "a_CoorSys_S[m|s2]"
  CUSTOM_POINTS_1/11 -> Bus Creator2/10  "Angle_Ver_CoorSys_S[deg]"
  CUSTOM_POINTS_1/8 -> Bus Creator2/7  "Pos_CoorSys_S[x;y;z][m]"
  CUSTOM_POINTS_1/9 -> Bus Creator2/8  "Pos_CoorSys_E[x;y;z][m]"
  CUSTOM_POINTS_1/15 -> Bus Creator2/14  "Data_4[]"
  CUSTOM_POINTS_1/16 -> Bus Creator2/15  "Data_5[]"
  CUSTOM_POINTS_1/14 -> Bus Creator2/13  "Data_3[]"
  CUSTOM_POINTS_1/2 -> Bus Creator2/1  "Flag_In_Scope[0|1]"
  CUSTOM_POINTS_1/6 -> Bus Creator2/5  "v_CoorSys_S[m|s]"
  CUSTOM_POINTS_1/17 -> Bus Creator2/16  "Object_ID[]"
  CUSTOM_POINTS_1/12 -> Bus Creator2/11  "Data_1[]"
  CUSTOM_POINTS_1/5 -> Bus Creator2/4  "Dist_CoorSys_S[m]"
  CUSTOM_POINTS_1/3 -> Bus Creator2/2  "Flag_Is_Occluded[0|1]"
  CUSTOM_POINTS_1/10 -> Bus Creator2/9  "Angle_Hor_CoorSys_S[deg]"
  CUSTOM_POINTS_1/4 -> Bus Creator2/3  "ID[]"
  CUSTOM_POINTS_1/13 -> Bus Creator2/12  "Data_2[]"
  Bus Creator2/1 -> CustomPoint_Signals[]/1
  CUSTOM_POINTS_1/1 -> Terminator/1
  Sensor_Idx[]/1 -> CUSTOM_POINTS_1/1
  Sensor_Data[]/1 -> CUSTOM_POINTS_1/2

== system ASM_Traffic_V2X_Complete_Model_2/MDL/Environment/Traffic/Sensors/Object_Sensor_3D/CustomPoints/Sensor1/CustomPointsOutput ==
  SensorSchedulingEnable[0|1] : Inport
  SensorActive[0|1] : Inport  Port=2
  SensorEnable[0|1] : Inport  Port=3
  DelayPulse[0|1] : Inport  Port=4
  CustomPoints_Signals_In[] : Inport  Port=5
  CUSTOM_POINTS_SIGNALS_DELAY_1 : ASM_Traffic_lib/Sensors/Custom Points/CUSTOM_POINTS_SIGNALS_DELAY  ASMProperties=struct('Name','CUSTOM_POINTS_SIGNALS_DELAY','Version','1.0','Library','ASM_Traffic_lib')  ASMInstanceName=custom_points_signals_delay  ASMInstanceID=1
  HoldSignals : Subsystem
  Logical Operator1 : Logic  Operator=OR  AllPortsSameDT=off  OutDataTypeStr=boolean
  ResetPulse : Subsystem
  SignalBus : Subsystem
  CustomPoints_Signals_Out[] : Outport
  wires:
  ResetPulse/1(ResetPulse[0|1]) -> Logical Operator1/1, HoldSignals/1(ResetPulse[0|1]), CUSTOM_POINTS_SIGNALS_DELAY_1/1
  SensorEnable[0|1]/1 -> Logical Operator1/2
  Logical Operator1/1 -> HoldSignals/Enable
  SensorActive[0|1]/1 -> ResetPulse/2(SensorActive[0|1])
  HoldSignals/1(CustomPoints_Signals_Out[]) -> CUSTOM_POINTS_SIGNALS_DELAY_1/3
  SignalBus/1(CustomPoints_Signals_Out[]) -> CustomPoints_Signals_Out[]/1
  DelayPulse[0|1]/1 -> CUSTOM_POINTS_SIGNALS_DELAY_1/2
  CUSTOM_POINTS_SIGNALS_DELAY_1/1 -> SignalBus/1(CustomPoints_Signals_In[])
  CustomPoints_Signals_In[]/1 -> HoldSignals/2(CustomPoints_Signals_In[])
  SensorSchedulingEnable[0|1]/1 -> ResetPulse/1(Enable[0|1])

== system ASM_Traffic_V2X_Complete_Model_2/MDL/Environment/Traffic/Sensors/Object_Sensor_3D/CustomPoints/Sensor2/CustomPoints ==
  Sensor_Idx[] : Inport
  Sensor_Data[] : Inport  Port=2
  Enable : EnablePort
  Bus Creator2 : BusCreator  Inputs=17
  CUSTOM_POINTS_2 : ASM_Traffic_lib/Sensors/Custom Points/CUSTOM_POINTS  Tag=ASM_SUBCOMPONENT  Sw_Visible_Points_Filter_Enable=MDL.Traffic.Sensors.CustomPoints_2.Sw_Visible_Points_Filter_Enable  Sw_Sort_Enable=MDL.Traffic.Sensors.CustomPoints_2.Sw_Sort_Enable  Sw_Sort_Attribute=MDL.Traffic.Sensors.CustomPoints_2.Sw_Sort_Attribute  Sw_Sort_Direction=MDL.Traffic.Sensors.CustomPoints_2.Sw_Sort_Direction  ASMProperties=struct('Name','CUSTOM_POINTS','Version','1.0','Library','ASM_Traffic_lib')  ASMInstanceName=custom_points  ASMInstanceID=2  Const_Output_Dimension_Objects=MDL.Traffic.Sensors.CustomPoints_2.Const_Output_Dimension_Objects  Const_Output_Dimension_Object_Points=MDL.Traffic.Sensors.CustomPoints_2.Const_Output_Dimension_Object_Points
      settings: AttributesFormatString=Instance Name: custom_points\nInstance ID: 2
  MODELDESK_GROUP : ASM_Utils_lib/ModelDeskInterface/MODELDESK_GROUP  MDLDGroup=Object Sensor 3D 2  ASMProperties=struct('Name','MODELDESK_GROUP','Version','1.0','Library','ASM_Utils_lib')
  Terminator : Terminator
  CustomPoint_Signals[] : Outport  OutputWhenDisabled=reset  InitialOutput=[0]
  wires:
  CUSTOM_POINTS_2/4 -> Bus Creator2/3  "ID[]"
  CUSTOM_POINTS_2/8 -> Bus Creator2/7  "Pos_CoorSys_S[x;y;z][m]"
  CUSTOM_POINTS_2/9 -> Bus Creator2/8  "Pos_CoorSys_E[x;y;z][m]"
  CUSTOM_POINTS_2/14 -> Bus Creator2/13  "Data_3[]"
  CUSTOM_POINTS_2/3 -> Bus Creator2/2  "Flag_Is_Occluded[0|1]"
  CUSTOM_POINTS_2/12 -> Bus Creator2/11  "Data_1[]"
  CUSTOM_POINTS_2/2 -> Bus Creator2/1  "Flag_In_Scope[0|1]"
  CUSTOM_POINTS_2/13 -> Bus Creator2/12  "Data_2[]"
  CUSTOM_POINTS_2/16 -> Bus Creator2/15  "Data_5[]"
  CUSTOM_POINTS_2/6 -> Bus Creator2/5  "v_CoorSys_S[m|s]"
  CUSTOM_POINTS_2/7 -> Bus Creator2/6  "a_CoorSys_S[m|s2]"
  CUSTOM_POINTS_2/11 -> Bus Creator2/10  "Angle_Ver_CoorSys_S[deg]"
  CUSTOM_POINTS_2/10 -> Bus Creator2/9  "Angle_Hor_CoorSys_S[deg]"
  CUSTOM_POINTS_2/5 -> Bus Creator2/4  "Dist_CoorSys_S[m]"
  CUSTOM_POINTS_2/15 -> Bus Creator2/14  "Data_4[]"
  CUSTOM_POINTS_2/17 -> Bus Creator2/16  "Object_ID[]"
  CUSTOM_POINTS_2/18 -> Bus Creator2/17  "Object_Type[]"
  Sensor_Data[]/1 -> CUSTOM_POINTS_2/2
  Sensor_Idx[]/1 -> CUSTOM_POINTS_2/1
  Bus Creator2/1 -> CustomPoint_Signals[]/1
  CUSTOM_POINTS_2/1 -> Terminator/1

== system ASM_Traffic_V2X_Complete_Model_2/MDL/Environment/Traffic/Sensors/Object_Sensor_3D/CustomPoints/Sensor2/CustomPointsOutput ==
  SensorSchedulingEnable[0|1] : Inport
  SensorActive[0|1] : Inport  Port=2
  SensorEnable[0|1] : Inport  Port=3
  DelayPulse[0|1] : Inport  Port=4
  CustomPoint_Signals_In[] : Inport  Port=5
  CUSTOM_POINTS_SIGNALS_DELAY_2 : ASM_Traffic_lib/Sensors/Custom Points/CUSTOM_POINTS_SIGNALS_DELAY  ASMProperties=struct('Name','CUSTOM_POINTS_SIGNALS_DELAY','Version','1.0','Library','ASM_Traffic_lib')  ASMInstanceName=custom_points_signals_delay  ASMInstanceID=1
  HoldSignals : Subsystem
  Logical Operator1 : Logic  Operator=OR  AllPortsSameDT=off  OutDataTypeStr=boolean
  ResetPulse : Subsystem
  SignalBus : Subsystem
  CustomPoints_Signals_Out[] : Outport
  wires:
  SensorActive[0|1]/1 -> ResetPulse/2(SensorActive[0|1])
  ResetPulse/1(ResetPulse[0|1]) -> Logical Operator1/1, HoldSignals/1(ResetPulse[0|1]), CUSTOM_POINTS_SIGNALS_DELAY_2/1
  SensorEnable[0|1]/1 -> Logical Operator1/2
  SensorSchedulingEnable[0|1]/1 -> ResetPulse/1(Enable[0|1])
  DelayPulse[0|1]/1 -> CUSTOM_POINTS_SIGNALS_DELAY_2/2
  Logical Operator1/1 -> HoldSignals/Enable
  HoldSignals/1(CustomPoints_Signals_Out[]) -> CUSTOM_POINTS_SIGNALS_DELAY_2/3
  SignalBus/1(CustomPoints_Signals_Out[]) -> CustomPoints_Signals_Out[]/1
  CUSTOM_POINTS_SIGNALS_DELAY_2/1 -> SignalBus/1(CustomPoints_Signals_In[])
  CustomPoint_Signals_In[]/1 -> HoldSignals/2(CustomPoints_Signals_In[])

== system ASM_Traffic_V2X_Complete_Model_2/MDL/Environment/Traffic/Sensors/Object_Sensor_3D/CustomPoints/Sensor3/CustomPoints ==
  Sensor_Idx[] : Inport
  Sensor_Data[] : Inport  Port=2
  Enable : EnablePort
  Bus Creator2 : BusCreator  Inputs=17
  CUSTOM_POINTS_3 : ASM_Traffic_lib/Sensors/Custom Points/CUSTOM_POINTS  Tag=ASM_SUBCOMPONENT  Sw_Visible_Points_Filter_Enable=MDL.Traffic.Sensors.CustomPoints_3.Sw_Visible_Points_Filter_Enable  Sw_Sort_Enable=MDL.Traffic.Sensors.CustomPoints_3.Sw_Sort_Enable  Sw_Sort_Attribute=MDL.Traffic.Sensors.CustomPoints_3.Sw_Sort_Attribute  Sw_Sort_Direction=MDL.Traffic.Sensors.CustomPoints_3.Sw_Sort_Direction  ASMProperties=struct('Name','CUSTOM_POINTS','Version','1.0','Library','ASM_Traffic_lib')  ASMInstanceName=custom_points  ASMInstanceID=3  Const_Output_Dimension_Objects=MDL.Traffic.Sensors.CustomPoints_3.Const_Output_Dimension_Objects  Const_Output_Dimension_Object_Points=MDL.Traffic.Sensors.CustomPoints_3.Const_Output_Dimension_Object_Points
      settings: AttributesFormatString=Instance Name: custom_points\nInstance ID: 3
  MODELDESK_GROUP : ASM_Utils_lib/ModelDeskInterface/MODELDESK_GROUP  MDLDGroup=Object Sensor 3D 3  ASMProperties=struct('Name','MODELDESK_GROUP','Version','1.0','Library','ASM_Utils_lib')
  Terminator : Terminator
  CustomPoint_Signals[] : Outport  OutputWhenDisabled=reset  InitialOutput=[0]
  wires:
  CUSTOM_POINTS_3/15 -> Bus Creator2/14  "Data_4[]"
  CUSTOM_POINTS_3/14 -> Bus Creator2/13  "Data_3[]"
  CUSTOM_POINTS_3/3 -> Bus Creator2/2  "Flag_Is_Occluded[0|1]"
  CUSTOM_POINTS_3/6 -> Bus Creator2/5  "v_CoorSys_S[m|s]"
  CUSTOM_POINTS_3/17 -> Bus Creator2/16  "Object_ID[]"
  CUSTOM_POINTS_3/13 -> Bus Creator2/12  "Data_2[]"
  CUSTOM_POINTS_3/4 -> Bus Creator2/3  "ID[]"
  CUSTOM_POINTS_3/10 -> Bus Creator2/9  "Angle_Hor_CoorSys_S[deg]"
  CUSTOM_POINTS_3/8 -> Bus Creator2/7  "Pos_CoorSys_S[x;y;z][m]"
  CUSTOM_POINTS_3/18 -> Bus Creator2/17  "Object_Type[]"
  CUSTOM_POINTS_3/2 -> Bus Creator2/1  "Flag_In_Scope[0|1]"
  CUSTOM_POINTS_3/11 -> Bus Creator2/10  "Angle_Ver_CoorSys_S[deg]"
  CUSTOM_POINTS_3/12 -> Bus Creator2/11  "Data_1[]"
  CUSTOM_POINTS_3/5 -> Bus Creator2/4  "Dist_CoorSys_S[m]"
  CUSTOM_POINTS_3/9 -> Bus Creator2/8  "Pos_CoorSys_E[x;y;z][m]"
  CUSTOM_POINTS_3/16 -> Bus Creator2/15  "Data_5[]"
  CUSTOM_POINTS_3/7 -> Bus Creator2/6  "a_CoorSys_S[m|s2]"
  Sensor_Idx[]/1 -> CUSTOM_POINTS_3/1
  Sensor_Data[]/1 -> CUSTOM_POINTS_3/2
  Bus Creator2/1 -> CustomPoint_Signals[]/1
  CUSTOM_POINTS_3/1 -> Terminator/1

== system ASM_Traffic_V2X_Complete_Model_2/MDL/Environment/Traffic/Sensors/Object_Sensor_3D/CustomPoints/Sensor3/CustomPointsOutput ==
  SensorSchedulingEnable[0|1] : Inport
  SensorActive[0|1] : Inport  Port=2
  SensorEnable[0|1] : Inport  Port=3
  DelayPulse[0|1] : Inport  Port=4
  CustomPoints_Signals_In[] : Inport  Port=5
  CUSTOM_POINTS_SIGNALS_DELAY_3 : ASM_Traffic_lib/Sensors/Custom Points/CUSTOM_POINTS_SIGNALS_DELAY  ASMProperties=struct('Name','CUSTOM_POINTS_SIGNALS_DELAY','Version','1.0','Library','ASM_Traffic_lib')  ASMInstanceName=custom_points_signals_delay  ASMInstanceID=1
  HoldSignals : Subsystem
  Logical Operator1 : Logic  Operator=OR  AllPortsSameDT=off  OutDataTypeStr=boolean
  ResetPulse1 : Subsystem
  SignalBus : Subsystem
  CustomPoints_Signals_Out[] : Outport
  wires:
  DelayPulse[0|1]/1 -> CUSTOM_POINTS_SIGNALS_DELAY_3/2
  SensorActive[0|1]/1 -> ResetPulse1/2(SensorActive[0|1])
  ResetPulse1/1(ResetPulse[0|1]) -> HoldSignals/1(ResetPulse[0|1]), Logical Operator1/1, CUSTOM_POINTS_SIGNALS_DELAY_3/1
  SensorSchedulingEnable[0|1]/1 -> ResetPulse1/1(Enable[0|1])
  SensorEnable[0|1]/1 -> Logical Operator1/2
  HoldSignals/1(CustomPoints_Signals_Out[]) -> CUSTOM_POINTS_SIGNALS_DELAY_3/3
  Logical Operator1/1 -> HoldSignals/Enable
  SignalBus/1(CustomPoints_Signals_Out[]) -> CustomPoints_Signals_Out[]/1
  CUSTOM_POINTS_SIGNALS_DELAY_3/1 -> SignalBus/1(CustomPoints_Signals_In[])
  CustomPoints_Signals_In[]/1 -> HoldSignals/2(CustomPoints_Signals_In[])
